simulink model "sm_boom_lift_damper_valve"  (R2026a)
settings: Solver=VariableStepAuto  StopTime=20
libraries: fl_lib x15, nesl_utility x10, Custom_Valves x2, MyMath_lib x1, simulink x1
Description:
  | Copyright 2020-2026 The MathWorks, Inc.
settings Model: Creator=smiller  LastModifiedBy=smiller
settings SimscapeCC: SimscapeNominalValues="[{\"value\":\"1\",\"unit\":\"A\"},{\"value\":\"nomval_psi\",\"unit\":\"psi\"},{\"value\":\"1\",\"unit\":\"cm^2\"},{\"value\":\"nomval_cmv3_s\",\"unit\":\"cm^3/s\"},{\"value\":\"1\",\"unit\":\"kJ/kg\"},{\"value\":\"1\",\"unit\":\"kW\"},{\"value\":\"1\",\"unit\":\"l\"},{\"value\":\"nomval_N\",\"unit\":\"N\"},{\"value\":\"nomval_Nm\",\"unit\":\"N*m\"},{\"value\":\"1\",\"unit\":\"V\"}]"  SimscapeLogDataHistory=5000.0

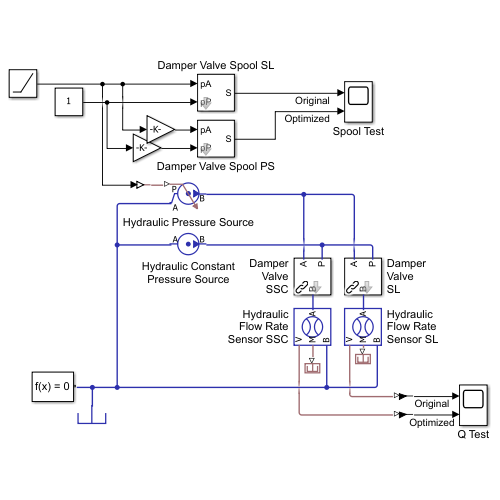
[thumbnail: Simulink's stored preview of the top-level diagram]
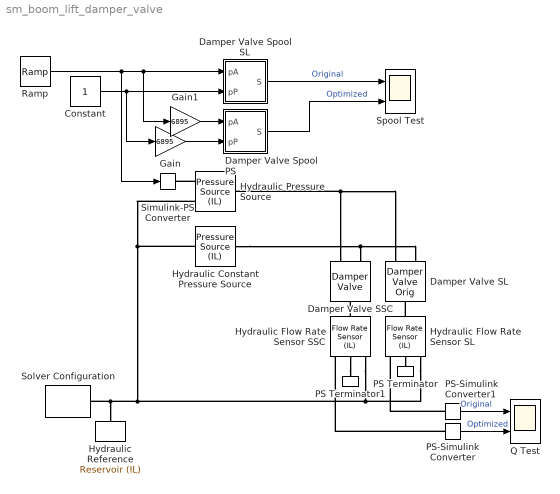
== system sm_boom_lift_damper_valve ==
  Constant : Constant
  Damper Valve SL : Custom_Valves/Damper Valve Orig  sMax=valves.control.l.max  T=2e-2  AMax=orifices.sky.d1.s  pCrack=25  pMax=75
  Damper Valve SSC : Custom_Valves/Damper Valve  sMax=valves.control.l.max  T=2e-2  AMax=orifices.sky.d1.s  pCrack=25  pMax=75
  Damper Valve Spool PS : Subsystem  mask{sMax=valves.control.l.max, T=2e-2, AMax=orifices.sky.d1.s, pCrack=25, pMax=75}
      mask prompts: sMax "Maximum Valve Opening, in"; T "First-Order Time Lag, s"; AMax "Maximum Passage Area, in^2"; pCrack "Cracking Pressure, PSI"; pMax "Maximum Pressure, PSI"
      mask init:
      | % Calculate spring rate, k, assuming that the valve spring is the only
      | % element used to control the valve opening:
      | k = (pMax - pCrack)/sMax;
  Damper Valve Spool SL : Subsystem  mask{sMax=valves.control.l.max, T=2e-2, AMax=orifices.sky.d1.s, pCrack=25, pMax=75}
      mask prompts: sMax "Maximum Valve Opening, in"; T "First-Order Time Lag, s"; AMax "Maximum Passage Area, in^2"; pCrack "Cracking Pressure, PSI"; pMax "Maximum Pressure, PSI"
      mask init:
      | % Calculate spring rate, k, assuming that the valve spring is the only
      | % element used to control the valve opening:
      | k = (pMax - pCrack)/sMax;
  Gain : Gain  Gain=6895
  Gain1 : Gain  Gain=6895
  Hydraulic Flow Rate Sensor SL : fl_lib/Isothermal Liquid/Sensors/Flow Rate Sensor (IL)  sensor_type=3
  Hydraulic Flow Rate Sensor SSC : fl_lib/Isothermal Liquid/Sensors/Flow Rate Sensor (IL)  sensor_type=3
  Hydraulic Constant Pressure Source : fl_lib/Isothermal Liquid/Sources/Pressure Source (IL)  source_type=1  pressure_differential=1 psi
  Hydraulic Pressure Source : fl_lib/Isothermal Liquid/Sources/Pressure Source (IL)  source_type=foundation.enum.constant_controlled.controlled  pressure_differential=0 MPa
  Hydraulic Reference : fl_lib/Isothermal Liquid/Elements/Reservoir (IL)  pressure_input=false  pressure_spec=foundation.enum.pressure_spec.atmospheric  reservoir_pressure=0.101325 MPa
  PS Terminator : fl_lib/Physical Signals/Sinks/PS Terminator
  PS Terminator1 : fl_lib/Physical Signals/Sinks/PS Terminator
  PS-Simulink Converter : nesl_utility/PS-Simulink Converter  PhysicalDomain=network_engine_domain  SubClassName=ps_output  LeftPortType=input  RightPortType=output  PseudoPeriodic=off  Frequencies=[]  VectorFormat=1-D array  Unit=inherit  AffineConversion=off
  PS-Simulink Converter1 : nesl_utility/PS-Simulink Converter  PhysicalDomain=network_engine_domain  SubClassName=ps_output  LeftPortType=input  RightPortType=output  PseudoPeriodic=off  Frequencies=[]  VectorFormat=1-D array  Unit=inherit  AffineConversion=off
  Q Test : Scope  NumInputPorts=2
      settings: Title=Flow Rate Test  ActiveDisplayYMinimum=-2E-6  ActiveDisplayYMaximum=1.5E-5
  Ramp : simulink/Sources/Ramp  slope=5  start=0  InitialOutput=20
  Simulink-PS Converter : nesl_utility/Simulink-PS Converter  PhysicalDomain=network_engine_domain  SubClassName=ps_input  LeftPortType=input  RightPortType=output  PseudoPeriodic=off  Frequencies=[]  NoiseDistribution=none  NoiseParameters=[]  Unit=psi  AffineConversion=off  FilteringAndDerivatives=provide  SimscapeFilterOrder=1  InputFilterTimeConstant=0.001  UdotUserProvided=0
  Solver Configuration : nesl_utility/Solver Configuration  PhysicalDomain=network_engine_domain  SubClassName=solver  LeftPortType=input  RightPortType=generic  Tones=[]  Harmonics=[]  SimulateNoise=off  Profile=off  UseLocalSampling=off  EnableSwitchedLinearOptims=on  FrequencyDomain=off  UseCCode=off  RelTol=0.001  AbsTol=1e-06  MinStep=1e-09  ToWorkspace=off  RevertToSquareIcSolve=off  NumHomotopyIterations=100  PhasorMode=off  PhasorModeNumHarmonics=1  ConsistencySolver=NEWTON_FTOL  CanonicalOrdering=UNORDERED  OptimizeIntermediates=UNOPTIMIZED  IndexReductionMethod=DerivativeReplacement  DoDC=off  ResidualTolerance=1e-09  ConsistencyTolSource=GLOBAL  ConsistencyAbsTol=0.001  ConsistencyRelTol=0.001  ConsistencyTolFactor=0.001  UseLocalSolver=off  LocalSolverChoice=NE_BACKWARD_EULER_ADVANCER  ResolveIndetEquations=on  FunctionEvalNumThread=1  LocalSolverSampleTime=0.001  DoFixedCost=off  MaxNonlinIter=3  MaxModeIter=2  ComputeImpulses=off  ImpulseIterations=2  LinearAlgebra=auto  LinearAlgebraNumThread=0  EquationFormulation=NE_TIME_EF  DelaysMemoryBudget=1024  AutomaticFiltering=on  FilteringTimeConstant=0.001  PartitionStorageMethod=AS_NEEDED  PartitionMemoryBudget=1024  PartitionMethod=ROBUST  MultibodyUseLocalSolver=off  MultibodyLocalSolverChoice=ODE1  MultibodyLocalSolverSampleTime=0.001
  Spool Test : Scope  NumInputPorts=2
      settings: Title=Spool Test  ActiveDisplayYMinimum=-0.125  ActiveDisplayYMaximum=1.125
  wires:
  Ramp/1 -> Simulink-PS Converter/1, Gain1/1, Damper Valve Spool SL/1(pA)
  Constant/1 -> Gain/1, Damper Valve Spool SL/2(pP)
  Damper Valve Spool SL/1(S) -> Spool Test/1  "Original"
  Damper Valve Spool PS/1(S) -> Spool Test/2  "Optimized"
  Gain/1 -> Damper Valve Spool PS/2(pP)
  Gain1/1 -> Damper Valve Spool PS/1(pA)
  PS-Simulink Converter/1 -> Q Test/2  "Optimized"
  PS-Simulink Converter1/1 -> Q Test/1  "Original"
  connections:
  Hydraulic Flow Rate Sensor SL/RConn2 -- PS Terminator/LConn1
  PS-Simulink Converter1/LConn1 -- Hydraulic Flow Rate Sensor SL/RConn3
  Hydraulic Flow Rate Sensor SSC/LConn1 -- Damper Valve SSC/RConn1
  Hydraulic Flow Rate Sensor SSC/RConn2 -- PS Terminator1/LConn1
  PS-Simulink Converter/LConn1 -- Hydraulic Flow Rate Sensor SSC/RConn3
  Damper Valve SSC/LConn1 -- Damper Valve SL/LConn1 -- Hydraulic Pressure Source/RConn1
  Hydraulic Pressure Source/LConn2 -- Simulink-PS Converter/RConn1
  Hydraulic Constant Pressure Source/RConn1 -- Damper Valve SL/LConn2 -- Damper Valve SSC/LConn2
  Hydraulic Reference/LConn1 -- Hydraulic Constant Pressure Source/LConn1 -- Hydraulic Pressure Source/LConn1 -- Hydraulic Flow Rate Sensor SSC/RConn1 -- Hydraulic Flow Rate Sensor SL/RConn1 -- Solver Configuration/RConn1
  Hydraulic Flow Rate Sensor SL/LConn1 -- Damper Valve SL/RConn1

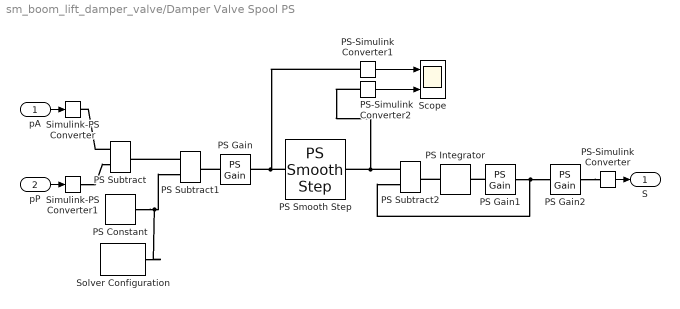
== system sm_boom_lift_damper_valve/Damper Valve Spool PS ==
  pA : Inport
  pP : Inport  Port=2
  PS Constant : fl_lib/Physical Signals/Sources/PS Constant  constant=pCrack*6895 Pa
  PS Gain : fl_lib/Physical Signals/Functions/PS Gain  gain=1/k*0.000145038 1/Pa
  PS Gain1 : fl_lib/Physical Signals/Functions/PS Gain  gain=1/T 1/s
  PS Gain2 : fl_lib/Physical Signals/Functions/PS Gain  gain=1 m^2
  PS Integrator : fl_lib/Physical Signals/Linear Operators/PS Integrator  reset_method=foundation.enum.IntegratorResetSpec.None  initial_condition_spec=foundation.enum.IntegratorICSpec.Internal  saturation_spec=foundation.enum.IntegratorSaturationSpec.None  saturation_source_spec=foundation.enum.IntegratorSaturationSourceSpec.Internal  x0=0*T s  xu=inf s  xl=-inf s
  PS Smooth Step : MyMath_lib/PS Smooth Step  step_start=0  step_finish=sMax  min_out=0  max_out=sMax
  PS Subtract : fl_lib/Physical Signals/Functions/PS Subtract
  PS Subtract1 : fl_lib/Physical Signals/Functions/PS Subtract
  PS Subtract2 : fl_lib/Physical Signals/Functions/PS Subtract
  PS-Simulink Converter : nesl_utility/PS-Simulink Converter  PhysicalDomain=network_engine_domain  SubClassName=ps_output  LeftPortType=input  RightPortType=output  PseudoPeriodic=off  Frequencies=[]  VectorFormat=1-D array  Unit=inherit  AffineConversion=off
  PS-Simulink Converter1 : nesl_utility/PS-Simulink Converter  PhysicalDomain=network_engine_domain  SubClassName=ps_output  LeftPortType=input  RightPortType=output  PseudoPeriodic=off  Frequencies=[]  VectorFormat=1-D array  Unit=inherit  AffineConversion=off
  PS-Simulink Converter2 : nesl_utility/PS-Simulink Converter  PhysicalDomain=network_engine_domain  SubClassName=ps_output  LeftPortType=input  RightPortType=output  PseudoPeriodic=off  Frequencies=[]  VectorFormat=1-D array  Unit=inherit  AffineConversion=off
  Scope : Scope  NumInputPorts=2
      settings: ActiveDisplayYMinimum=-0.37001  ActiveDisplayYMaximum=2.13008
  Simulink-PS Converter : nesl_utility/Simulink-PS Converter  PhysicalDomain=network_engine_domain  SubClassName=ps_input  LeftPortType=input  RightPortType=output  PseudoPeriodic=off  Frequencies=[]  NoiseDistribution=none  NoiseParameters=[]  Unit=Pa  AffineConversion=off  FilteringAndDerivatives=provide  SimscapeFilterOrder=1  InputFilterTimeConstant=0.001  UdotUserProvided=0
  Simulink-PS Converter1 : nesl_utility/Simulink-PS Converter  PhysicalDomain=network_engine_domain  SubClassName=ps_input  LeftPortType=input  RightPortType=output  PseudoPeriodic=off  Frequencies=[]  NoiseDistribution=none  NoiseParameters=[]  Unit=Pa  AffineConversion=off  FilteringAndDerivatives=provide  SimscapeFilterOrder=1  InputFilterTimeConstant=0.001  UdotUserProvided=0
  Solver Configuration : nesl_utility/Solver Configuration  PhysicalDomain=network_engine_domain  SubClassName=solver  LeftPortType=input  RightPortType=generic  Tones=[]  Harmonics=[]  SimulateNoise=off  Profile=off  UseLocalSampling=off  EnableSwitchedLinearOptims=on  FrequencyDomain=off  UseCCode=off  RelTol=0.001  AbsTol=1e-06  MinStep=1e-09  ToWorkspace=off  RevertToSquareIcSolve=off  NumHomotopyIterations=100  PhasorMode=off  PhasorModeNumHarmonics=1  ConsistencySolver=NEWTON_FTOL  CanonicalOrdering=UNORDERED  OptimizeIntermediates=UNOPTIMIZED  IndexReductionMethod=DerivativeReplacement  DoDC=off  ResidualTolerance=1e-09  ConsistencyTolSource=GLOBAL  ConsistencyAbsTol=0.001  ConsistencyRelTol=0.001  ConsistencyTolFactor=0.001  UseLocalSolver=off  LocalSolverChoice=NE_BACKWARD_EULER_ADVANCER  ResolveIndetEquations=on  FunctionEvalNumThread=1  LocalSolverSampleTime=0.001  DoFixedCost=off  MaxNonlinIter=3  MaxModeIter=2  ComputeImpulses=off  ImpulseIterations=2  LinearAlgebra=auto  LinearAlgebraNumThread=0  EquationFormulation=NE_TIME_EF  DelaysMemoryBudget=1024  AutomaticFiltering=on  FilteringTimeConstant=0.001  PartitionStorageMethod=AS_NEEDED  PartitionMemoryBudget=1024  PartitionMethod=ROBUST  MultibodyUseLocalSolver=off  MultibodyLocalSolverChoice=ODE1  MultibodyLocalSolverSampleTime=0.001
  S : Outport
  wires:
  pP/1 -> Simulink-PS Converter1/1
  pA/1 -> Simulink-PS Converter/1
  PS-Simulink Converter/1 -> S/1
  PS-Simulink Converter1/1 -> Scope/1
  PS-Simulink Converter2/1 -> Scope/2
  connections:
  PS Subtract/LConn1 -- Simulink-PS Converter/RConn1
  Simulink-PS Converter1/RConn1 -- PS Subtract/LConn2
  PS Subtract1/LConn1 -- PS Subtract/RConn1
  PS Gain/LConn1 -- PS Subtract1/RConn1
  PS Constant/RConn1 -- Solver Configuration/RConn1 -- PS Subtract1/LConn2
  PS Smooth Step/LConn1 -- PS-Simulink Converter1/LConn1 -- PS Gain/RConn1
  PS Gain2/RConn1 -- PS-Simulink Converter/LConn1
  PS Subtract2/LConn1 -- PS-Simulink Converter2/LConn1 -- PS Smooth Step/RConn1
  PS Integrator/LConn1 -- PS Subtract2/RConn1
  PS Gain1/LConn1 -- PS Integrator/RConn1
  PS Gain1/RConn1 -- PS Subtract2/LConn2 -- PS Gain2/LConn1

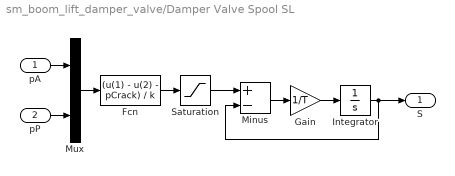
== system sm_boom_lift_damper_valve/Damper Valve Spool SL ==
  pA : Inport
  pP : Inport  Port=2
  Fcn : Fcn  Expr=(u(1) - u(2) - pCrack) / k
  Gain : Gain  Gain=1/T
  Integrator : Integrator
  Minus : Sum  Inputs=+-
  Mux : Mux  Inputs=2
  Saturation : Saturate  UpperLimit=sMax  LowerLimit=0
  S : Outport
  wires:
  Integrator/1 -> S/1, Minus/2
  Gain/1 -> Integrator/1
  Minus/1 -> Gain/1
  Saturation/1 -> Minus/1
  Mux/1 -> Fcn/1
  pA/1 -> Mux/1
  pP/1 -> Mux/2
  Fcn/1 -> Saturation/1
